simulink model "Q5"  (R2015a)
settings: Solver=ode45  StartTime=0.0  StopTime=10.0  RelTol=1e-3
values from neighbouring files (symbols this model uses):
  cte1 = (beta) / ( ((M*(L^2))/3) + m*(l^2) )    (= 2.24719101124)    [lab3.m]
  cte2 = ( m*g*l + (M*g*L/2) -k ) / ( ((M*(L^2))/3) + m*(l^2) )    (= -41.5393258427)    [lab3.m]
  teta0 = pi/4    (= 0.785398163397)    [lab3.m]
  U = 0    [lab3.m]
  v0 = 0    [lab3.m]
settings Model: Creator=Diogo  LastModifiedBy=Diogo

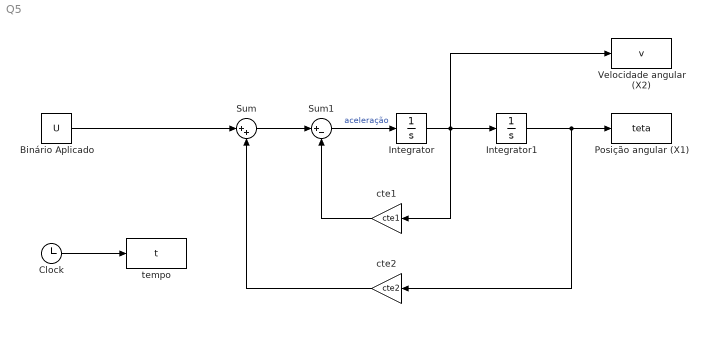
== system Q5 ==
  Binário Aplicado : Constant  Value=U
  Clock : Clock
  Integrator : Integrator  InitialCondition=v0
  Integrator1 : Integrator  InitialCondition=teta0
  Posição angular (X1) : ToWorkspace  VariableName=teta  SampleTime=0.01
  Sum : Sum  Inputs=|++
  Sum1 : Sum  Inputs=|+-
  Velocidade angular (X2) : ToWorkspace  VariableName=v  SampleTime=0.01
  cte1 : Gain  Gain=cte1
  cte2 : Gain  Gain=cte2
  tempo : ToWorkspace  VariableName=t  SampleTime=0.01
  wires:
  Sum/1 -> Sum1/1
  cte1/1 -> Sum1/2
  cte2/1 -> Sum/2
  Sum1/1 -> Integrator/1  "aceleração"
  Binário Aplicado/1 -> Sum/1
  Integrator1/1 -> Posição angular (X1)/1, cte2/1
  Clock/1 -> tempo/1
  Integrator/1 -> Integrator1/1, cte1/1, Velocidade angular (X2)/1
